simulink model "physicalmotortest"  (R2020b)
settings: Solver=FixedStepAuto  StartTime=0.0  StopTime=inf  FixedStep=0.1  RelTol=1e-3  EnableMultiTasking=on
libraries: arduinolib x6, simulink x1
settings Model: SILPILModeSetting=veronly  ExtModeTrigDuration=2  Creator=Ege  LastModifiedBy=Ege
settings OptimizationCC: EnhancedBackFolding=on  PassReuseOutputArgsAs=Individual arguments  ZeroExternalMemoryAtStartup=off  ZeroInternalMemoryAtStartup=off  MaxStackSize=64  OptimizeBlockOrder=speed  DifferentSizesBufferReuse=on  OptimizationCustomize=off  EfficientTunableParamExpr=on
settings DebuggingCC: ParameterTunabilityLossMsg=error
settings HardwareCC: ProdBitPerPointer=32  ProdBitPerSizeT=32  ProdBitPerPtrDiffT=32  ProdLargestAtomicInteger=Long  ProdLargestAtomicFloat=Double  ProdWordSize=32  ProdHWDeviceType=ARM Compatible->ARM Cortex
settings SFSimCC: MATLABDynamicMemAlloc=off
settings RTWCC: Description=Embedded Coder  SystemTargetFile=ert.tlc  HardwareBoard=Arduino Nano 33 IoT  TemplateMakefile=ert_default_tmf  Toolchain=Arduino ARM  BuildConfiguration=Faster Runs
settings CodeAppCC: ForceParamTrailComments=on  IgnoreCustomStorageClasses=off  OperatorAnnotations=on  SimulinkDataObjDesc=on  SFDataObjDesc=on  InsertBlockDesc=on
settings ERTTargetCC: SupportContinuousTime=on  SupportVariableSizeSignals=on  ExtModeTransport=3  ExtModeStaticAllocSize=8192  ExtModeMexFile=ext_xcp  ExtModeIntrfLevel=Level2 - Open

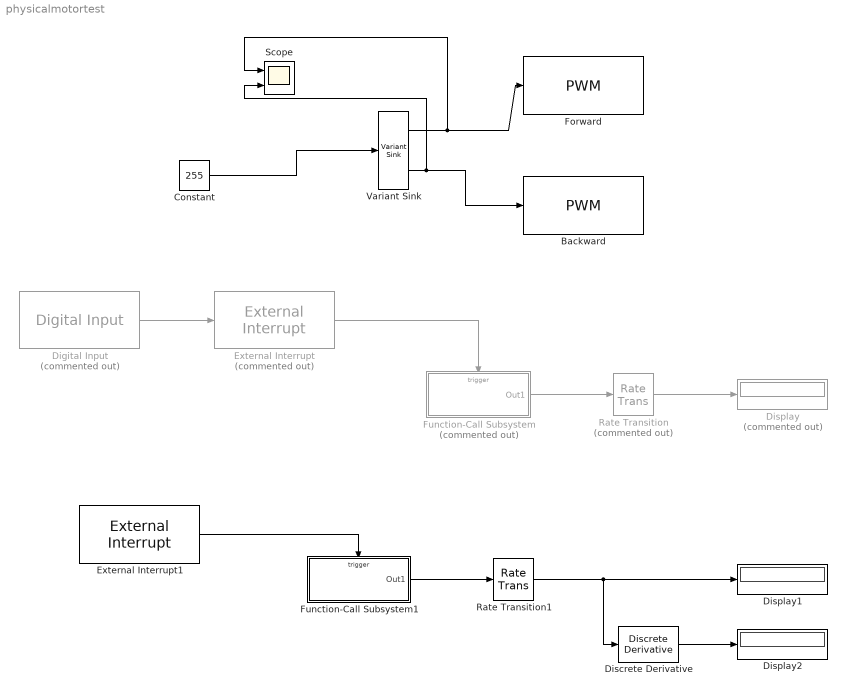
== system physicalmotortest ==
  Backward : arduinolib/PWM  pinNumber=11  frequencyType=Default  desiredFrequency=490.2  achievableFrequency=490.2
  Constant : Constant  Value=255  SampleTime=-1
  Digital Input : arduinolib/Digital Input  Commented=on  pinNumber=3  mode=Default  Direction=input  SampleTime=-1  blockPlatform=arduino
  Discrete Derivative : simulink/Discrete/Discrete Derivative  gainval=1.0  ICPrevScaledInput=0.0  OutMin=[]  OutMax=[]  OutDataType=fixdt(1, 16)  OutScaling=2^-10  DoSatur=off
  Display : Display  Commented=on
  Display1 : Display
  Display2 : Display
  External Interrupt : arduinolib/External Interrupt  Commented=on  Pin=2  PullUp=off  Mode=RISING  InterruptSimulationInput=on
      settings: SourceProductBaseCode=ARDUINO
  External Interrupt1 : arduinolib/External Interrupt  Pin=2  PullUp=off  Mode=RISING  InterruptSimulationInput=off
      settings: SourceProductBaseCode=ARDUINO
  Forward : arduinolib/PWM  pinNumber=10  frequencyType=Default  desiredFrequency=490.2  achievableFrequency=490.2
  Function-Call Subsystem : Subsystem  Commented=on  TreatAsAtomicUnit=on
  Function-Call Subsystem1 : Subsystem  TreatAsAtomicUnit=on
  Rate Transition : RateTransition  Commented=on  Deterministic=off
  Rate Transition1 : RateTransition  Deterministic=off
  Scope : Scope  NumInputPorts=2
  Variant Sink : VariantSink
  wires:
  Variant Sink/2 -> Scope/2, Backward/1
  Constant/1 -> Variant Sink/1
  Variant Sink/1 -> Scope/1, Forward/1
  External Interrupt/1 -> Function-Call Subsystem/Trigger
  Function-Call Subsystem/1(Out1) -> Rate Transition/1
  Rate Transition/1 -> Display/1
  Digital Input/1 -> External Interrupt/1
  Rate Transition1/1 -> Discrete Derivative/1, Display1/1
  Function-Call Subsystem1/1(Out1) -> Rate Transition1/1
  External Interrupt1/1 -> Function-Call Subsystem1/Trigger
  Discrete Derivative/1 -> Display2/1

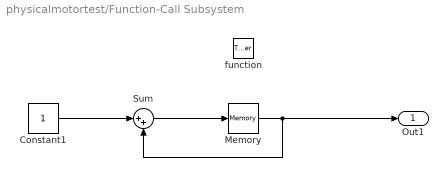
== system physicalmotortest/Function-Call Subsystem ==
  function : TriggerPort  TriggerType=function-call  VariantControl=Variant  SampleTime=-1
  Constant1 : Constant
  Memory : Memory  InheritSampleTime=on
  Sum : Sum  Inputs=|++
  Out1 : Outport
  wires:
  Memory/1 -> Out1/1, Sum/2
  Sum/1 -> Memory/1
  Constant1/1 -> Sum/1

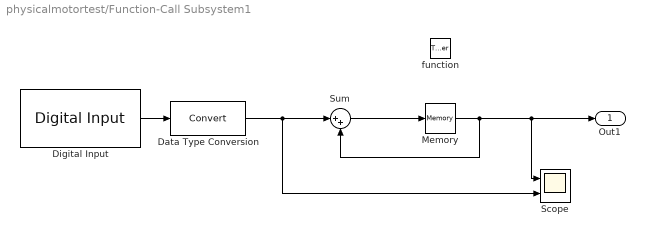
== system physicalmotortest/Function-Call Subsystem1 ==
  function : TriggerPort  TriggerType=function-call  VariantControl=Variant  SampleTime=-1
  Data Type Conversion : DataTypeConversion
  Digital Input : arduinolib/Digital Input  pinNumber=3  mode=Default  Direction=input  SampleTime=-1  blockPlatform=arduino
  Memory : Memory  InheritSampleTime=on
  Scope : Scope  NumInputPorts=2
  Sum : Sum  Inputs=|++
  Out1 : Outport
  wires:
  Memory/1 -> Scope/1, Out1/1, Sum/2
  Sum/1 -> Memory/1
  Digital Input/1 -> Data Type Conversion/1
  Data Type Conversion/1 -> Scope/2, Sum/1
